simulink model "bike_to_line"  (R2022b)
settings: Solver=VariableStepAuto  StartTime=0.0  StopTime=20  RelTol=1e-3
model workspace (MAT data in the model file):
  L = 1
  La = 1
  Lb = -2
  Lc = 4
  xo = [8 5 1.57079632679]
undefined symbols (not defined in the file): magnitude
libraries: simulink x1
settings Model: Creator=cesguti  LastModifiedBy=cesguti

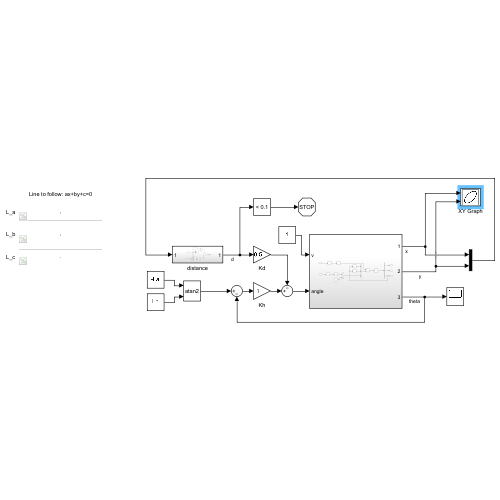
[thumbnail: Simulink's stored preview of the top-level diagram]
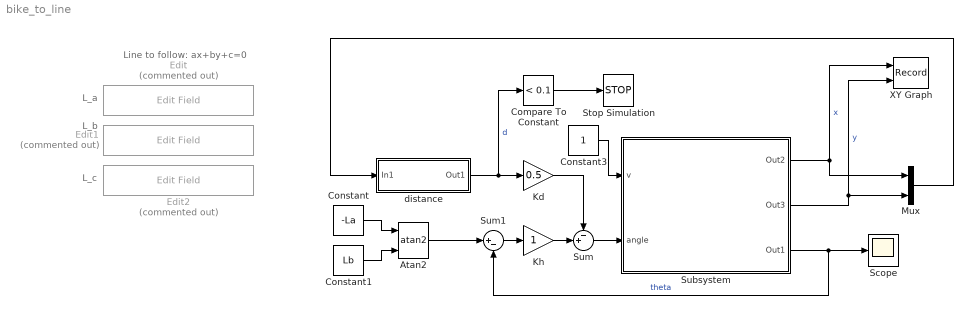
== system bike_to_line ==
  note: Line to follow: ax+by+c=0
  note: L_a
  note: L_b
  note: L_c
  Atan2 : Trigonometry  Operator=atan2
  Compare To Constant : simulink/Logic and Bit Operations/Compare To Constant  relop=<  const=0.1  OutDataTypeStr=boolean
  Constant : Constant  Value=-La
  Constant1 : Constant  Value=Lb
  Constant3 : Constant
  Edit : EditField  Commented=on  LabelPosition=Hide  ShowInitialText=on  Alignment=Center
  Edit1 : EditField  Commented=on  LabelPosition=Hide  ShowInitialText=on  Alignment=Center
  Edit2 : EditField  Commented=on  LabelPosition=Hide  ShowInitialText=on  Alignment=Center
  Kd : Gain  Gain=0.5
  Kh : Gain
  Mux : Mux  Inputs=2
  Scope : Scope
  Stop Simulation : Stop
  Subsystem : Subsystem
  Sum : Sum  Inputs=-+|
  Sum1 : Sum  Inputs=|+-
  XY Graph : Record  FileSettingsInternal="{\"entries\":[{\"content\":{\"excelSettings\":{\"content\":{},\"type\":\"Streamout.ExcelSettings\"}},\"type\":\"Streamout.FileSettingStorage\",\"uuid\":\"ccbf8a72-8350-462c-9974-8677f415f9db\"}],\"packageUris\":[\"http://schema.mathworks.com/mf0/streamout_blocks/R2020a\"],\"version\":\"1.0\"}"  Layout=[1 1]  SignalsInternal="{\"entries\":[{\"content\":{\"signals\":[{\"content\":{\"blockPath\":[\"bike_to_line/XY Graph\"],\"channel\":[],\"dimensions\":[1],\"domain\":\"bike_to_line/XY Graph\",\"lineColor\":\"#a2142f\",\"plots\":[1],\"port\":1,\"sid\":[\"\"],\"signalID\":2107,\"signalName\":\"x\"},\"type\":\"RecordBlkView.Signal\",\"uuid\":\"2edb2a56-079f-4da2-a096-56302438d940\"},{\"content\":{\"blockPath\":[\"bike_to_line/XY Graph\"],\"channel\":[],\"dimensions\":[1],\"domain\":\"bike_to_line/XY Graph\",\"lineColor\":\"#139fff\",\"plots\":[1],\"port\":2,\"sid\":[\"\"],\"signalID\":2111,\"signalName\":\"y\"},\"type\":\"RecordBlkView.Signal\",\"uuid\":\"2e118317-c19b-463f-9934-facdc5d2f9b9\"}]},\"type\":\"RecordBlkView.InputSignals\",\"uuid\":\"41025663-227e-438b-ab95-4cab457e7d5c\"}],\"packageUris\":[\"http://schema.mathworks.com/mf0/streamout_blocks/R2020a\"],\"version\":\"1.0\"}"  VisualizationBindings="{\"xyplotplugin\":{\"info\":[{\"series\":[{\"bindingParametersList\":[{\"parameter\":\"X-Axis\",\"signalID\":2107,\"signalName\":\"x\"},{\"parameter\":\"Y-Axis\",\"signalID\":2111,\"signalName\":\"y\"}],\"seriesID\":32726}],\"subplotID\":1}]}}"  CompatibilityTag=XY
  distance : Subsystem
  wires:
  distance/1(Out1) -> Compare To Constant/1, Kd/1  "d"
  Sum1/1 -> Kh/1
  Subsystem/1(Out2) -> XY Graph/1, Mux/1  "x"
  Subsystem/2(Out3) -> XY Graph/2, Mux/2  "y"
  Atan2/1 -> Sum1/1
  Subsystem/3(Out1) -> Scope/1, Sum1/2  "theta"
  Compare To Constant/1 -> Stop Simulation/1
  Kh/1 -> Sum/2
  Sum/1 -> Subsystem/2(angle)
  Kd/1 -> Sum/1
  Constant3/1 -> Subsystem/1(v)
  Constant/1 -> Atan2/1
  Constant1/1 -> Atan2/2
  Mux/1 -> distance/1(In1)

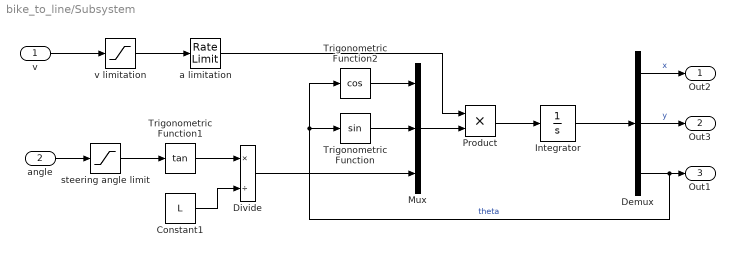
== system bike_to_line/Subsystem ==
  v : Inport
  angle : Inport  Port=2
  Constant1 : Constant  Value=L
  Demux : Demux  Outputs=3
  Divide : Product  Inputs=*/
  Integrator : Integrator  InitialCondition=xo
  Mux : Mux  Inputs=3
  Product : Product
  Trigonometric Function : Trigonometry
  Trigonometric Function1 : Trigonometry  Operator=tan
  Trigonometric Function2 : Trigonometry  Operator=cos
  a limitation : RateLimiter  SampleTimeMode=inherited
  steering angle limit : Saturate  UpperLimit=deg2rad(60)  LowerLimit=deg2rad(-60)
  v limitation : Saturate  UpperLimit=1  LowerLimit=0
  Out2 : Outport
  Out3 : Outport  Port=2
  Out1 : Outport  Port=3
  wires:
  steering angle limit/1 -> Trigonometric Function1/1
  Product/1 -> Integrator/1
  Divide/1 -> Mux/3
  Trigonometric Function/1 -> Mux/2
  v/1 -> v limitation/1
  Constant1/1 -> Divide/2
  Mux/1 -> Product/2
  Trigonometric Function1/1 -> Divide/1
  Trigonometric Function2/1 -> Mux/1
  v limitation/1 -> a limitation/1
  Integrator/1 -> Demux/1
  angle/1 -> steering angle limit/1
  Demux/3 -> Out1/1, Trigonometric Function/1, Trigonometric Function2/1  "theta"
  a limitation/1 -> Product/1
  Demux/1 -> Out2/1  "x"
  Demux/2 -> Out3/1  "y"

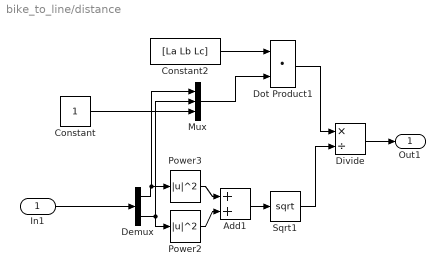
== system bike_to_line/distance ==
  In1 : Inport
  Add1 : Sum
  Constant : Constant
  Constant2 : Constant  Value=[La Lb Lc]
  Demux : Demux  Outputs=2
  Divide : Product  Inputs=*/
  Dot Product1 : DotProduct  OutDataTypeStr=Inherit: Inherit via internal rule
  Mux : Mux  Inputs=3
  Power2 : Math  Operator=magnitude^2
  Power3 : Math  Operator=magnitude^2
  Sqrt1 : Sqrt
  Out1 : Outport
  wires:
  In1/1 -> Demux/1
  Constant2/1 -> Dot Product1/1
  Demux/1 -> Mux/1, Power3/1
  Demux/2 -> Mux/2, Power2/1
  Power3/1 -> Add1/1
  Power2/1 -> Add1/2
  Add1/1 -> Sqrt1/1
  Divide/1 -> Out1/1
  Sqrt1/1 -> Divide/2
  Dot Product1/1 -> Divide/1
  Mux/1 -> Dot Product1/2
  Constant/1 -> Mux/3
